simulink model "MRACDireto_Gradiente_Deducao_Winnie"  (R2015a)
settings: Solver=ode1  StartTime=0.0  StopTime=20  FixedStep=1e-4  RelTol=1e-3
undefined symbols (not defined in the file): b, gamma, it, ref
settings Model: Creator=user  LastModifiedBy=user

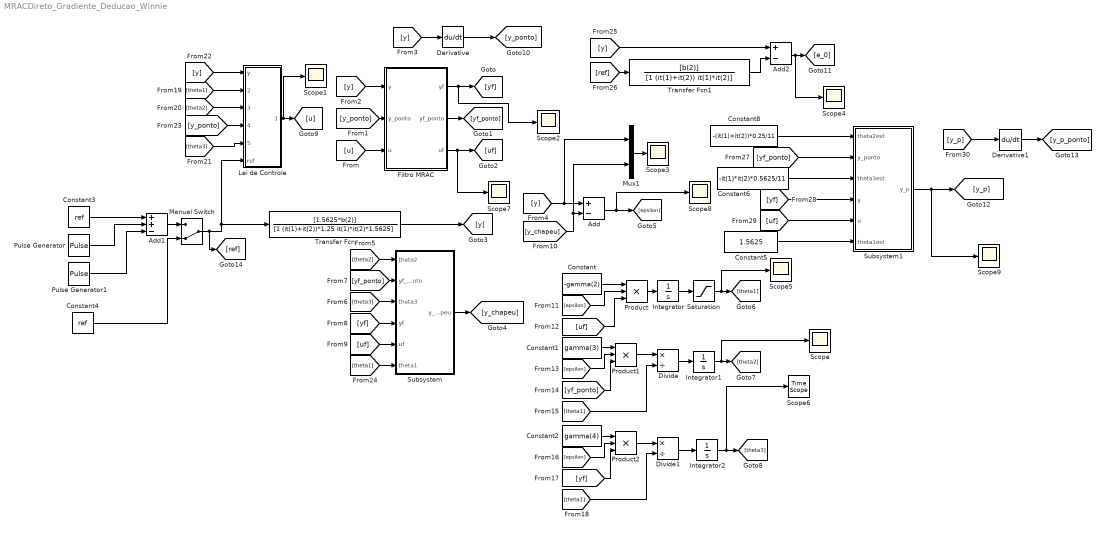
== system MRACDireto_Gradiente_Deducao_Winnie ==
  Add : Sum  Inputs=+-
  Add1 : Sum  Inputs=++-
  Add2 : Sum  Inputs=+-
  Constant : Constant  Value=-gamma(2)
  Constant1 : Constant  Value=gamma(3)
  Constant2 : Constant  Value=gamma(4)
  Constant3 : Constant  Value=ref
  Constant4 : Constant  Value=ref
  Constant5 : Constant  Value=1.5625
  Constant6 : Constant  Value=-it(1)*it(2)*0.5625/11
  Constant8 : Constant  Value=-(it(1)+it(2))*0.25/11
  Derivative : Derivative
  Derivative1 : Derivative
  Divide : Product  Inputs=*/
  Divide1 : Product  Inputs=*/
  "Filtro MRAC " : Subsystem
  Integrator : Integrator  InitialCondition=0.1
  Integrator1 : Integrator  InitialCondition=-0.20
  Integrator2 : Integrator  InitialCondition=-0.2
  Lei de Controle : Subsystem
  Manual Switch : ManualSwitch  CurrentSetting=0
  Mux1 : Mux  Inputs=2
  Product : Product  Inputs=3
  Product1 : Product  Inputs=3
  Product2 : Product  Inputs=3
  Pulse Generator : DiscretePulseGenerator  PulseType=Time based  Amplitude=ref/40  Period=1  PulseWidth=5
  Pulse Generator1 : DiscretePulseGenerator  PulseType=Time based  Amplitude=ref/40  PulseWidth=50
  Saturation : Saturate  UpperLimit=92347563487568273465  LowerLimit=0.1
  Scope{,1..5,7..9} (9 alike) : Scope
      Scope settings: YMin=0.7795  YMax=0.7825
      Scope1 settings: TimeRange=300  YMin=0  YMax=110
      Scope2 settings: TimeRange=1  YMin=50.143  YMax=50.1431  SaveName=ScopeData2
      Scope3 settings: TimeRange=1  YMin=110  YMax=110  SaveName=ScopeData3
      Scope4 settings: TimeRange=20  YMin=-8.67362e-19  YMax=0.025  SaveName=ScopeData4
      Scope5 settings: YMin=0.115  YMax=0.1425  SaveName=ScopeData5
      Scope7 settings: TimeRange=1  YMin=50.143  YMax=50.1431  SaveName=ScopeData7
      Scope8 settings: TimeRange=1  YMin=7.5e-06  YMax=2.75e-05  SaveName=ScopeData8
      Scope9 settings: TimeRange=60  YMin=-0.2  YMax=0  SaveName=ScopeData9
  Scope6 : TimeScope
  Subsystem : Subsystem
  Subsystem1 : Subsystem
  Transfer Fcn : TransferFcn  Numerator=[1.5625*b(2)]  Denominator=[1 (it(1)+it(2))*1.25 it(1)*it(2)*1.5625]
  Transfer Fcn1 : TransferFcn  Numerator=[b(2)]  Denominator=[1 (it(1)+it(2)) it(1)*it(2)]
  wires:
  [y] -> "Filtro MRAC "/1(y)
  [y_ponto] -> "Filtro MRAC "/2(y_ponto)
  [u] -> "Filtro MRAC "/3(u)
  "Filtro MRAC "/3(uf) -> Scope7/1, [uf]
  [theta2] -> Subsystem/1(theta2)
  [yf_ponto] -> Subsystem/2(yf_ponto)
  [theta3] -> Subsystem/3(theta3)
  [yf] -> Subsystem/4(yf)
  [uf] -> Subsystem/5(uf)
  Subsystem/1(y_chapeu) -> [y_chapeu]
  [y] -> Mux1/1, Add/1
  [y_chapeu] -> Mux1/2, Add/2
  Add/1 -> Scope8/1, [epsilon]
  Constant/1 -> Product/1
  [epsilon] -> Product/2
  [uf] -> Product/3
  Product/1 -> Integrator/1
  Constant1/1 -> Product1/1
  [epsilon] -> Product1/2
  [yf_ponto] -> Product1/3
  Integrator1/1 -> Scope/1, [theta2]
  Product1/1 -> Divide/1
  Divide/1 -> Integrator1/1
  [theta1] -> Divide/2
  Integrator/1 -> Saturation/1
  [epsilon] -> Product2/2
  [yf] -> Product2/3
  Integrator2/1 -> Scope6/1, [theta3]
  Product2/1 -> Divide1/1
  Divide1/1 -> Integrator2/1
  [theta1] -> Divide1/2
  Constant2/1 -> Product2/1
  [y] -> Lei de Controle/1(y)
  [theta1] -> Lei de Controle/2(theta1)
  [theta2] -> Lei de Controle/3(theta2)
  [y_ponto] -> Lei de Controle/4(yponto)
  [theta3] -> Lei de Controle/5(theta3)
  Lei de Controle/1(Out1) -> Scope1/1, [u]
  Mux1/1 -> Scope3/1
  [y] -> Derivative/1
  Derivative/1 -> [y_ponto]
  Saturation/1 -> Scope5/1, [theta1]
  "Filtro MRAC "/2(yf_ponto) -> [yf_ponto]
  "Filtro MRAC "/1(yf) -> Scope2/1, [yf]
  [theta1] -> Subsystem/6(theta1)
  Constant3/1 -> Add1/1
  Pulse Generator/1 -> Add1/2
  Pulse Generator1/1 -> Add1/3
  Add1/1 -> Manual Switch/1
  Manual Switch/1 -> [ref], Transfer Fcn/1, Lei de Controle/6(ref)
  Constant4/1 -> Manual Switch/2
  Transfer Fcn/1 -> [y]
  Add2/1 -> Scope4/1, [e_0]
  [y] -> Add2/1
  Transfer Fcn1/1 -> Add2/2
  [ref] -> Transfer Fcn1/1
  [uf] -> Subsystem1/5(u)
  [yf] -> Subsystem1/4(y)
  [yf_ponto] -> Subsystem1/2(y_ponto)
  Subsystem1/1(y_p) -> [y_p], Scope9/1
  [y_p] -> Derivative1/1
  Derivative1/1 -> [y_p_ponto]
  Constant5/1 -> Subsystem1/6(theta1est)
  Constant6/1 -> Subsystem1/3(theta3est)
  Constant8/1 -> Subsystem1/1(theta2est)

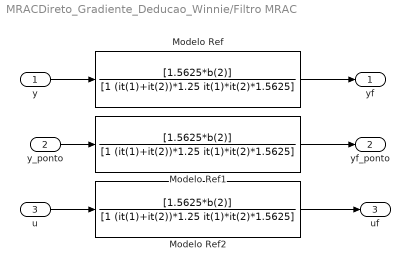
== system MRACDireto_Gradiente_Deducao_Winnie/Filtro MRAC  ==
  y : Inport
  y_ponto : Inport  Port=2
  u : Inport  Port=3
  Modelo Ref : TransferFcn  Numerator=[1.5625*b(2)]  Denominator=[1 (it(1)+it(2))*1.25 it(1)*it(2)*1.5625]
  Modelo Ref1 : TransferFcn  Numerator=[1.5625*b(2)]  Denominator=[1 (it(1)+it(2))*1.25 it(1)*it(2)*1.5625]
  Modelo Ref2 : TransferFcn  Numerator=[1.5625*b(2)]  Denominator=[1 (it(1)+it(2))*1.25 it(1)*it(2)*1.5625]
  yf : Outport
  yf_ponto : Outport  Port=2
  uf : Outport  Port=3
  wires:
  u/1 -> Modelo Ref2/1
  Modelo Ref2/1 -> uf/1
  y/1 -> Modelo Ref/1
  y_ponto/1 -> Modelo Ref1/1
  Modelo Ref/1 -> yf/1
  Modelo Ref1/1 -> yf_ponto/1

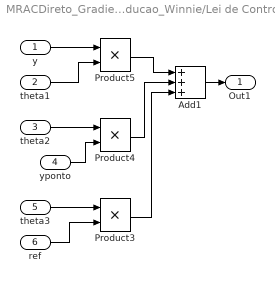
== system MRACDireto_Gradiente_Deducao_Winnie/Lei de Controle ==
  y : Inport
  theta1 : Inport  Port=2
  theta2 : Inport  Port=3
  yponto : Inport  Port=4
  theta3 : Inport  Port=5
  ref : Inport  Port=6
  Add1 : Sum  Inputs=+++
  Product3 : Product
  Product4 : Product
  Product5 : Product
  Out1 : Outport
  wires:
  Add1/1 -> Out1/1
  theta3/1 -> Product3/1
  theta2/1 -> Product4/1
  yponto/1 -> Product4/2
  Product3/1 -> Add1/3
  Product5/1 -> Add1/1
  theta1/1 -> Product5/2
  Product4/1 -> Add1/2
  y/1 -> Product5/1
  ref/1 -> Product3/2

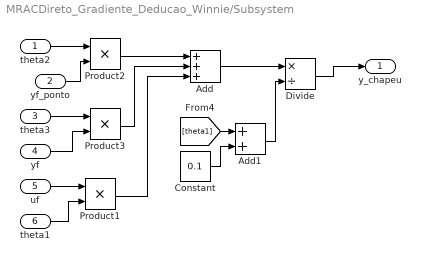
== system MRACDireto_Gradiente_Deducao_Winnie/Subsystem ==
  theta2 : Inport
  yf_ponto : Inport  Port=2
  theta3 : Inport  Port=3
  yf : Inport  Port=4
  uf : Inport  Port=5
  theta1 : Inport  Port=6
  Add : Sum  Inputs=+++
  Add1 : Sum
  Constant : Constant  Value=0.1
  Divide : Product  Inputs=*/
  Product1 : Product
  Product2 : Product
  Product3 : Product
  y_chapeu : Outport
  wires:
  Product3/1 -> Add/2
  theta2/1 -> Product2/1
  yf/1 -> Product3/2
  theta3/1 -> Product3/1
  Product2/1 -> Add/1
  Divide/1 -> y_chapeu/1
  Add/1 -> Divide/1
  yf_ponto/1 -> Product2/2
  [theta1] -> Add1/1
  Add1/1 -> Divide/2
  Constant/1 -> Add1/2
  uf/1 -> Product1/1
  theta1/1 -> Product1/2
  Product1/1 -> Add/3

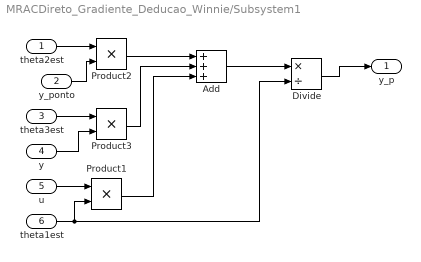
== system MRACDireto_Gradiente_Deducao_Winnie/Subsystem1 ==
  theta2est : Inport
  y_ponto : Inport  Port=2
  theta3est : Inport  Port=3
  y : Inport  Port=4
  u : Inport  Port=5
  theta1est : Inport  Port=6
  Add : Sum  Inputs=+++
  Divide : Product  Inputs=*/
  Product1 : Product
  Product2 : Product
  Product3 : Product
  y_p : Outport
  wires:
  Product1/1 -> Add/3
  u/1 -> Product1/1
  theta1est/1 -> Divide/2, Product1/2
  y_ponto/1 -> Product2/2
  Add/1 -> Divide/1
  Divide/1 -> y_p/1
  Product2/1 -> Add/1
  theta3est/1 -> Product3/1
  y/1 -> Product3/2
  theta2est/1 -> Product2/1
  Product3/1 -> Add/2
